simulink model "fss_2016a"  (R2016a)
settings: Solver=FixedStepAuto  SolverMode=SingleTasking  StartTime=0.0  StopTime=t(end)  FixedStep=dt  RelTol=1e-3
values from neighbouring files (symbols this model uses):
  Ab = -a_0*T*eye(3)    [isol_run.m]
  Asd = sysd.A    [isol_run.m]
  Bb = T*eye(3)    [isol_run.m]
  Bsd = sysd.B    [isol_run.m]
  Cb = (b_0-a_0*b_1)*H    [isol_run.m]
  Csd = sysd.C    [isol_run.m]
  Db = b_1*H    [isol_run.m]
  Dsd = sysd.D    [isol_run.m]
  dt = 0.005    [earthquake_select.m]    (also in isol_run.m)
  GL = zeros(1,lim-1);GL(1)=-alpha    [isol_run.m]
  Reduce = zeros(3,54);Reduce(:,49:51)=eye(3)    [isol_run.m]
  UL = Nt-1    [isol_run.m]
  xb_initial = zeros(3,1)    [isol_run.m]
  xs_initial = zeros(54,1)    [isol_run.m]
settings Model: Creator=tujia  LastModifiedBy=li2920
settings DebuggingCC: SFUnexpectedBacktrackingDiag=error  SFNoUnconditionalDefaultTransitionDiag=error
settings GRTTargetCC: TargetLangStandard=C99 (ISO)  GeneratePreprocessorConditionals=Use local settings
settings ConfigComp: CovMetricSettings=dwe  CovHtmlReporting=off  CovSaveCumulativeToWorkspaceVar=off  CovSaveSingleToWorkspaceVar=off  CovExternalEMLEnable=on

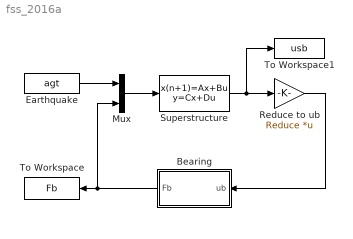
== system fss_2016a ==
  Bearing : Subsystem
  Earthquake : FromWorkspace  VariableName=agt  SampleTime=0
  Mux : Mux  Inputs=2
  Reduce to ub : Gain  Gain=Reduce  Multiplication=Matrix(K*u)
  Superstructure : DiscreteStateSpace  A=Asd  B=Bsd  C=Csd  D=Dsd  X0=xs_initial  SampleTime=dt
  To Workspace : ToWorkspace  VariableName=Fb  SaveFormat=Timeseries  SampleTime=dt
      settings: Save2DSignal=2-D array (concatenate along first dimension)
  To Workspace1 : ToWorkspace  VariableName=usb  SaveFormat=Timeseries  SampleTime=dt
      settings: Save2DSignal=2-D array (concatenate along first dimension)
  wires:
  Reduce to ub/1 -> Bearing/1(ub)
  Mux/1 -> Superstructure/1
  Superstructure/1 -> Reduce to ub/1, To Workspace1/1
  Earthquake/1 -> Mux/1
  Bearing/1(Fb) -> Mux/2, To Workspace/1

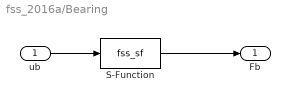
== system fss_2016a/Bearing ==
  ub : Inport
  S-Function : S-Function  FunctionName=fss_sf  Parameters=UL,GL,Ab,Bb,Cb,Db,xb_initial  SFunctionDeploymentMode=off  EnableBusSupport=off
  Fb : Outport
  wires:
  ub/1 -> S-Function/1
  S-Function/1 -> Fb/1
